simulink library "LumArduino"  (R2024a)
settings: Solver=VariableStepAuto  StartTime=0.0  StopTime=10.0  RelTol=1e-3
settings Model: Creator=chris  LastModifiedBy=chris

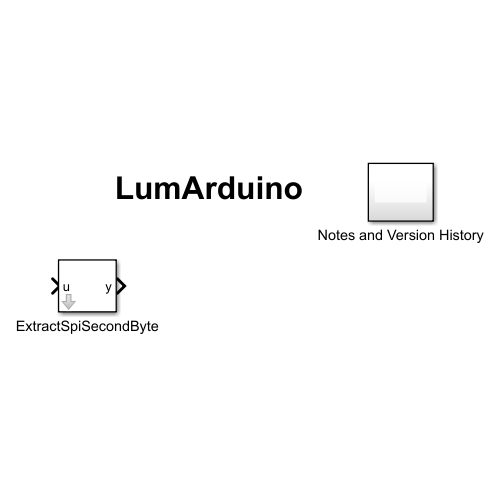
[thumbnail: Simulink's stored preview of the top-level diagram]
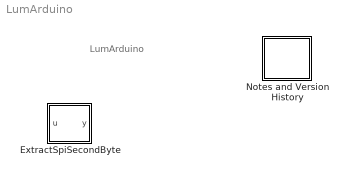
== system LumArduino ==
  note: LumArduino
  ExtractSpiSecondByte : Subsystem
      mask help:
      | An SPI WriteRead will likely involve the transfer of 2 bytes (the first being the address and the second being a dummy byte to obtain the data in the resulting duplex transfer).  Often the second returned byte is of interest and the first should be discarded.  This block extracts the desired second byte.
      |
      | Christopher Lum
      | lum@uw.edu
  Notes and Version History : Subsystem

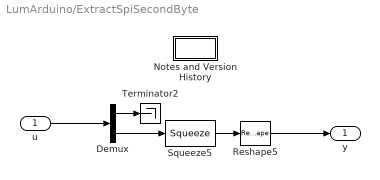
== system LumArduino/ExtractSpiSecondByte ==
  u : Inport
  Demux : Demux  Outputs=2
  Notes and Version History : Subsystem
  Reshape5 : Reshape
  Squeeze5 : Squeeze
  Terminator2 : Terminator
  y : Outport
  wires:
  u/1 -> Demux/1
  Demux/1 -> Terminator2/1
  Demux/2 -> Squeeze5/1
  Squeeze5/1 -> Reshape5/1
  Reshape5/1 -> y/1

== system LumArduino/Notes and Version History ==
  note: Various blocks and functionality to work with Arduino.
      |
      | Christopher Lum
      | lum@uw.edu
      |
      | Version History
      | 01/05/25: Created

== system LumArduino/ExtractSpiSecondByte/Notes and Version History ==
  note: Christopher Lum
      | lum@uw.edu
      |
      | Version History
      | 01/05/25: Created
